simulink model "sgMdl_IO141_AnalogDigitalLoopback"  (R2024b)
settings: Solver=FixedStepAuto  StartTime=0.0  StopTime=inf  RelTol=1e-3  EnableMultiTasking=on
libraries: speedgoatlib_IO141 x5
Description:
  | IO141 - Analog and Digital Loopback
settings Model: ModifiedByFormat=Speedgoat  SimulationMode=external  ExtModeEnableFloating=off  ExtModeTrigDuration=100000  Creator=Speedgoat  LastModifiedBy=Speedgoat
settings SolverCC: ConcurrentTasks=on  AlgebraicLoopSolver=TrustRegion  PositivePriorityOrder=on
settings DataIOCC: SaveFormat=StructureWithTime  ReturnWorkspaceOutputs=off
settings OptimizationCC: BlockReduction=off  OptimizeBlockIOStorage=off  BufferReuse=off  GlobalBufferReuse=off  ExpressionFolding=off  LocalBlockOutputs=off
settings DebuggingCC: TasksWithSamePriorityMsg=none  UnconnectedInputMsg=warning  UnconnectedOutputMsg=warning  UnconnectedLineMsg=warning  SFExecutionAtInitializationDiag=none  ArithmeticOperatorsInVariantConditions=warning
settings HardwareCC: ProdBitPerLong=64  ProdLongLongMode=on  ProdHWDeviceType=Intel->x86-64 (Linux 64)
settings ModelReferenceCC: EnableRefExpFcnMdlSchedulingChecks=on
settings SFSimCC: SimUseLocalCustomCode=off  CustomCodeUndefinedFunction=UseInterfaceOnly
settings RTWCC: Description=Speedgoat Real-Time Target Machine  SystemTargetFile=speedgoat.tlc  TemplateMakefile=slrealtime_default_tmf  RTWUseLocalCustomCode=off  Toolchain=Simulink Real-Time Toolchain  BuildConfiguration=Faster Runs  TargetLang=C++  GPUComputeCapability=3.5  DLArmComputeVersion=19.05
settings CodeAppCC: StateflowObjectComments=on
settings SimulinkRealTimeTargetCC: SubcomponentCodeInterfacePackaging=Reusable function  InstructionSetFMA=off  LogToMDFFile=off  SLRTFileLogMaxRuns=10  UseGCCFastMath=on
settings ConfigComp: CovBoundaryAbsTol=1.0e-5
settings SimscapeCC: SimscapeNormalizeSystem=off

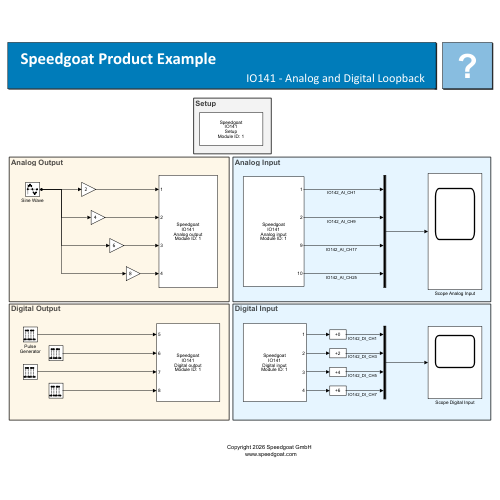
[thumbnail: Simulink's stored preview of the top-level diagram]
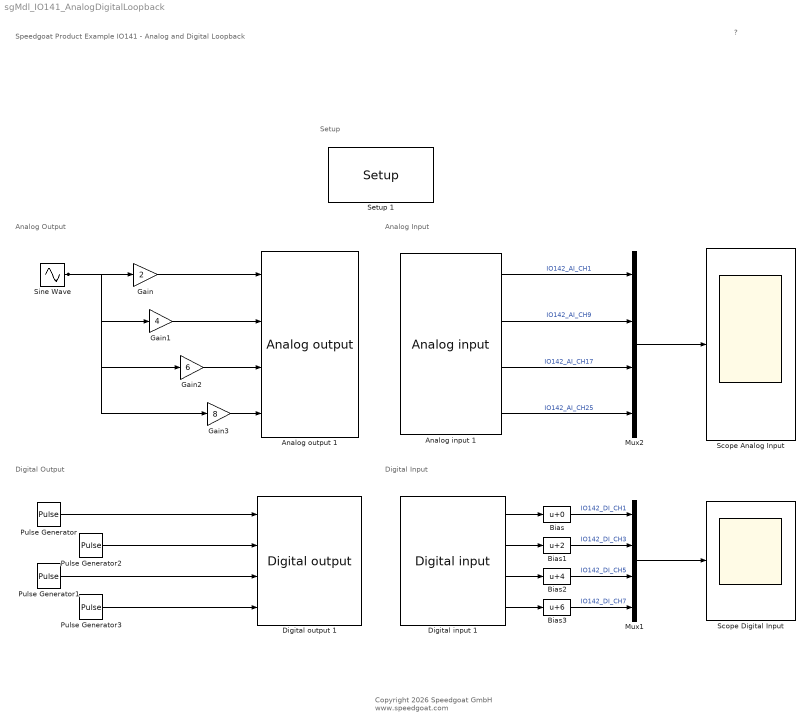
== system sgMdl_IO141_AnalogDigitalLoopback ==
  note: Analog Input
  note: Analog Output
  note: Digital Input
  note: Digital Output
  note: Setup
  note: Speedgoat Product Example
      | IO141 - Analog and Digital Loopback
  note: ?
  note: Copyright 2026 Speedgoat GmbH
      |  www.speedgoat.com
  Analog input 1 : speedgoatlib_IO141/Analog input   parModuleId=1  parSampleTime=0.001  parPciSlot=-1  parAdcChannels=[1 2 9 10]  parAdcNumActiveChannels=[2 2]  parAdcVoltageRange=[1 1 1 1 1 1 1 1 5 5 5 5 5 5 5 5]  parAdcCoupling=[1 1]  parAdcContSampling=0  parAdcDmaEnable=0  parAdcActiveDmaDevices=[1 1 1 1]  parAdcFrameSize=100
      settings: SourceProductName=Simulink Real-Time: Speedgoat I/O Blockset
  Analog output 1 : speedgoatlib_IO141/Analog output   parModuleId=1  parSampleTime=0.001  parPciSlot=-1  parDacChannels=[1 2 3 4]  parDacVoltageRange=[7 1 1 1]  parDacOverRange=[0 0 0 0]  parDacInitValues=[0 0 0 0]  parDacReset=[1 1 1 1]  parDacSyncOut=1  parDacDmaEnable=0  parDacActiveDmaDevices=[1 1 1 1]  parDacDmaLatency=2  parDacFrameSize=100
      settings: SourceProductName=Simulink Real-Time: Speedgoat I/O Blockset
  Bias : Bias  SaturateOnIntegerOverflow=off
  Bias1 : Bias  Bias=2  SaturateOnIntegerOverflow=off
  Bias2 : Bias  Bias=4  SaturateOnIntegerOverflow=off
  Bias3 : Bias  Bias=6  SaturateOnIntegerOverflow=off
  Digital input 1 : speedgoatlib_IO141/Digital input   parModuleId=1  parSampleTime=0.001  parPciSlot=-1  parDiChannels=[1 3 5 7]
      settings: SourceProductName=Simulink Real-Time: Speedgoat I/O Blockset
  Digital output 1 : speedgoatlib_IO141/Digital output   parModuleId=1  parSampleTime=0.001  parPciSlot=-1  parDoChannels=[2 4 6 8]  parDoInitValues=[0 0 0 0]  parDoReset=[1 1 1 1]
      settings: SourceProductName=Simulink Real-Time: Speedgoat I/O Blockset
  Gain : Gain  Gain=2
  Gain1 : Gain  Gain=4
  Gain2 : Gain  Gain=6
  Gain3 : Gain  Gain=8
  Mux1 : Mux
  Mux2 : Mux
  Pulse Generator : DiscretePulseGenerator  Period=25  PulseWidth=5  SampleTime=0.001
  Pulse Generator1 : DiscretePulseGenerator  Period=25  PulseWidth=15  SampleTime=0.001
  Pulse Generator2 : DiscretePulseGenerator  Period=25  PulseWidth=10  SampleTime=0.001
  Pulse Generator3 : DiscretePulseGenerator  Period=25  PulseWidth=20  SampleTime=0.001
  Scope Analog Input : Scope
  Scope Digital Input : Scope
  Setup 1 : speedgoatlib_IO141/Setup   parPciSlot=-1  parModuleId=1  parInterModuleSync=Independent  parConvClockBaseRate=20MHz  parConvClock1Divider=20000  parConvClock2Divider=20000  parFrameTriggerEnable=off  parFrameTriggerDivider=10  parConvClock1BaseRate=1  parConvClock2BaseRate=1  parFrameTriggerClock=1  parAdcCoupling1=Differential  parAdcChannels1=[1 2]  parAdcChannel11=on  parAdcChannel12=on  parAdcChannel13=off  parAdcChannel14=off  parAdcChannel15=off  parAdcChannel16=off  parAdcChannel17=off  parAdcChannel18=off  parAdcRangeAll1=+-0.64 V  parVoltageRangePerChannelEn1=off  parAdcRange11=+-0.64 V  parAdcRange12=+-0.64 V  parAdcRange13=+-0.64 V  parAdcRange14=+-0.64 V  parAdcRange15=+-0.64 V  parAdcRange16=+-0.64 V  parAdcRange17=+-0.64 V  parAdcRange18=+-0.64 V  parAdcCoupling2=Differential  parAdcChannels2=[9 10]  parAdcChannel21=on  parAdcChannel22=on  parAdcChannel23=off  parAdcChannel24=off  parAdcChannel25=off  parAdcChannel26=off  parAdcChannel27=off  parAdcChannel28=off  parAdcRangeAll2=+-10.24 V  parVoltageRangePerChannelEn2=off  parAdcRange21=+-0.64 V  parAdcRange22=+-0.64 V  parAdcRange23=+-0.64 V  parAdcRange24=+-0.64 V  parAdcRange25=+-0.64 V  parAdcRange26=+-0.64 V  parAdcRange27=+-0.64 V  parAdcRange28=+-0.64 V  parAdcChannels=[1 2 9 10]  parAdcNumActiveChannels=[2 2]  parAdcVoltageRange=[1 1 1 1 1 1 1 1 5 5 5 5 5 5 5 5]  parAdcCoupling=[1 1]  parAdcContSampling=off  parAdcAutoCorrection=on  parAdcDmaEnable=off  parAdcDmaClock=Clock 1  parAdcFrameSize_=100  parAdcSampleTime_=-1  parAdcActiveDmaDevices=[1 1 1 1]  parAdcFrameTriggerEnable=0  parAdcFrameSize=100  parAdcSampleTime=0.1  parDacChannels=[1 2]  parDacChannel1=on  parDacChannel2=on  parDacChannel3=on  parDacChannel4=on  parDacInitValues=0  parDacResets=1  parDacVoltageRange=[7 1 1 1]  parDacOverRange=[0 0 0 0]  parDacRange1=+-10 V  parDacInitValue1=0  parDacReset1=on  parDacRange2=0-5 V  parDacInitValue2=0  parDacReset2=on  parDacRange3=0-5 V  parDacInitValue3=0  parDacReset3=on  parDacRange4=0-5 V  parDacInitValue4=0  parDacReset4=on  parDacAutoCorrection=on  parDacSyncOut=on  parDacDmaEnable=off  parDacDmaLatency=Until next frame  parDacDmaClock=Clock 1  parDacFrameSize_=100  parDacSampleTime_=-1  parDacActiveDmaDevices=[1 1 1 1]  parDacFrameTriggerEnable=0  parDacFrameSize=100  parDacSampleTime=0.1  parDiChannels=[1 3 5 7]  parDoChannels=[2 4 6 8]  parDioChannel1=In  parDioChannel2=Out  parDioChannel3=In  parDioChannel4=Out  parDioChannel5=In  parDioChannel6=Out  parDioChannel7=In  parDioChannel8=Out  parDoInitValues=[0 0 0 0]  parDoReset=[1 1 1 1]  parDoInitValue1=0  parDoReset1=on  parDoInitValue2=0  parDoReset2=on  parDoInitValue3=0  parDoReset3=on  parDoInitValue4=0  parDoReset4=on  parDoInitValue5=0  parDoReset5=on  parDoInitValue6=0  parDoReset6=on  parDoInitValue7=0  parDoReset7=on  parDoInitValue8=0  parDoReset8=on  parDiDebounceEnable=off  parDiDebounceTime=0  parDiDebounceValue=0  parDioPullRefFront=Pull-up 3.3 V  parDioPullRefRear=Floating
      settings: SourceProductName=Simulink Real-Time: Speedgoat I/O Blockset
  Sine Wave : Sin  SineType=Sample based  Frequency=2*pi*5  Samples=50  SampleTime=0.001
  wires:
  Gain/1 -> Analog output 1/1
  Gain3/1 -> Analog output 1/4
  Sine Wave/1 -> Gain3/1, Gain2/1, Gain1/1, Gain/1
  Analog input 1/2 -> Mux2/2  "IO142_AI_CH9"
  Analog input 1/1 -> Mux2/1  "IO142_AI_CH1"
  Analog input 1/4 -> Mux2/4  "IO142_AI_CH25"
  Analog input 1/3 -> Mux2/3  "IO142_AI_CH17"
  Gain2/1 -> Analog output 1/3
  Gain1/1 -> Analog output 1/2
  Pulse Generator3/1 -> Digital output 1/4
  Pulse Generator1/1 -> Digital output 1/3
  Pulse Generator2/1 -> Digital output 1/2
  Pulse Generator/1 -> Digital output 1/1
  Mux1/1 -> Scope Digital Input/1
  Bias/1 -> Mux1/1  "IO142_DI_CH1"
  Bias1/1 -> Mux1/2  "IO142_DI_CH3"
  Bias2/1 -> Mux1/3  "IO142_DI_CH5"
  Bias3/1 -> Mux1/4  "IO142_DI_CH7"
  Mux2/1 -> Scope Analog Input/1
  Digital input 1/1 -> Bias/1
  Digital input 1/2 -> Bias1/1
  Digital input 1/3 -> Bias2/1
  Digital input 1/4 -> Bias3/1
